simulink model "ltao_e2e"  (R2022b)
settings: Solver=FixedStepDiscrete  StartTime=0.0  StopTime=30  FixedStep=FEM_Ts  MaxStep=FEM_Ts  RelTol=1e-2
InitFcn:
  | %
  | % Initialization callback function
  | %
  | 
  | try
  |    fprintf('\nGMT IMS version (%s)!\n',simulink_fname );
  | 
  |    % Get Simulink model directory
  |    [filepath,name,ext] = fileparts(which(bdroot));
  | 
  |    if ~strcmp(filepath,pwd)
  |       fprintf('\nChanging current directory to \n %s \n',filepath);
  |       cd(filepath);
  |    end
  | 
  |    %
  |  if(osim.bpless_wl)
  |     fprintf('Generating bumpless wind load time series\n');
  |  end
  | catch
  |    warning('Running the InitFcn from puSimulate script');
  | end
values from neighbouring files (symbols this model uses):
  asm_kl_dist = 0*asm_kl_dist    [load_ltao_e2e.m]
  asm_ssG = XiKL' * asm_ssG * XiKL    [load_ltao_e2e.m]
  Cpi_d = eye(n_Zmodes)* c2d(st.asm.fpi, Ts, c2d_opts)    [evalM2asm_modal.m]    (also in load_ltao_e2e.m = c2d(st.asm.fpi, FEM_Ts, c2d_opts))
  fao_d = c2d(st.glao.fao, st.glao.T, c2d_opts)    [evalM2asm_modal.m]    (also in load_ltao_e2e.m = c2d(st.ltao.fao, FEM_Ts, c2d_opts))
  fao_d4k = c2d(st.ltao.fao, 1/4e3, c2d_opts)    [evalM2asm_modal.m]    (also in load_ltao_e2e.m = c2d(st.ltao.fao, FEM_Ts, c2d_opts))
  FEM_Ts = 1/8e3    (= 0.000125)    [load_ltao_e2e.m]
  fes = c2d(tf((fc_es^2)*4*(pi^2),[1, 2*0.8*fc_es*2*pi, (fc_es^2)*4*(pi^2)]),     st.ltao.T,c2d_opts)    [load_ltao_e2e.m]
  flag_1stOdyn_d = tf(c2d(flag(2,1), Ts, c2d_opts))    [evalM2asm_modal.m]    (also in load_ltao_e2e.m = tf(c2d(flag(2,1),FEM_Ts,c2d_opts)))
  flag_2ndOdyn_d = tf(c2d(flag(3,1), Ts, c2d_opts))    [evalM2asm_modal.m]    (also in load_ltao_e2e.m = tf(c2d(flag(3,1),FEM_Ts,c2d_opts)))
  fm2off = c2d(f_ct_m2off, st.ltao.T,c2d_opts)    [load_ltao_e2e.m]
  fpre_d = tf(c2d(st.asm.fpre, Ts, c2d_opts))    [evalM2asm_modal.m]    (also in load_ltao_e2e.m = tf(c2d(fpre,FEM_Ts,c2d_opts)))
  gtt2mnt = eye(2)/(rbm2gtt * Hk_mnt_m1m2)    [load_ltao_e2e.m]
  Hk_mnt_m1m2 = Cm1m2*pinv(Cmnt)    [load_ltao_e2e.m]
  Hpd_d = eye(n_Zmodes)* c2d(st.asm.fpd, Ts, c2d_opts)    [evalM2asm_modal.m]    (also in load_ltao_e2e.m = c2d(st.asm.fpd, FEM_Ts, 'Tustin'))
  K_asm_2_m2p = K_m2p / K_m2p6F_2_asmRB    [load_ltao_e2e.m]
  K_m2p = gainMatrix(out_m2p_mc,in_m2p_mc) -gainMatrix(out_m2p_mc,in_m2p_m2)          - gainMatrix(out_m2p_m2,in_m2p_mc) +gainMatrix(out_m2p_m2,in_m2p_m2)    [load_ltao_e2e.m]
  K_m2p6F_2_asmRB = gainMatrix(out_asm_RB,in_m2p_mc) - gainMatrix(out_asm_RB,in_m2p_m2)    [load_ltao_e2e.m]
  K_m2p_2_asm = K_m2p6F_2_asmRB/ K_m2p    [load_ltao_e2e.m]
  K_m2p_2_es = gainMatrix(out_m2es,in_m2p_mc)-gainMatrix(out_m2es,in_m2p_m2)    [load_ltao_e2e.m]
  Kasmoff = K_asm_2_m2p *         [Kasmoff_{1},Kasmoff_{2},Kasmoff_{3},Kasmoff_{4},         Kasmoff_{5},Kasmoff_{6},Kasmoff_{7}]    [load_ltao_e2e.m]
  Ki_m2off = 1.3    [load_ltao_e2e.m]
  Km1rbm_es = (KhpF2es/KhpF2m1rbm)    [load_ltao_e2e.m]
  Ks = cell(7,1)    [load_ltao_e2e.m]
  m1_rbm_dist = zeros(42,1)    [load_ltao_e2e.m]
  m2_rbm_dist = 0*m2_rbm_dist    [load_ltao_e2e.m]
  m2_rbm_offset = 0*m2_rbm_offset    [load_ltao_e2e.m]
  PG = zeros(length(om2),6)    [evalM2asm_modal.m]    (also in load_ltao_e2e.m)
  phiB = inputs2ModalF(mode_ind_vec,indDesInputs) * KinputT    [load_ltao_e2e.m]
  phiC = KoutputT * modalDisp2Outputs(indDesOutputs,mode_ind_vec)    [load_ltao_e2e.m]
  Psi_ss = KoutputT *gainMatrix(indDesOutputs,indDesInputs)* KinputT - K_ss    [load_ltao_e2e.m]
  Rm2es = pinv(K_asm_2_es, 1e-2)    [load_ltao_e2e.m]
  segPTT2asmCMD = cell(7,1)    [load_ltao_e2e.m]
  st = getcontrol_asm()    [evalM2asm_modal.m]    (also in load_ltao_e2e.m)
  T_pos2e = (K_m2p_2_es / K_m2p)    [load_ltao_e2e.m]
undefined symbols (not defined in the file or in its folder): a, az, az_ff_en, b, c, D_seg_piston, D_seg_tt, DiscIntNeverNeededParam, el, fem, gir, m1sys, m2pos, magnitude, mount, osim, rbm2gtt, Rm1es, sm, VC_modal_stiff
libraries: ims_block_library x7, simulink x2
(part 1 of 3)
settings Model: SimulationMode=accelerator  Creator=RRomano  LastModifiedBy=rromano
settings SolverCC: MaxConsecutiveMinStep=10  ZeroCrossAlgorithm=Adaptive  AlgebraicLoopSolver=TrustRegion
settings DataIOCC: SaveOutput=off  SignalLogging=off  DSMLogging=off  SaveTime=off  ReturnWorkspaceOutputs=off
settings OptimizationCC: DefaultParameterBehavior=Inlined  StrengthReduction=on  PassReuseOutputArgsAs=Individual arguments  EfficientMapNaN2IntZero=off  SimCompilerOptimization=on  AccelVerboseBuild=on  OptimizeBlockOrder=speed  OptimizationPriority=Speed  OptimizationCustomize=off  MultiThreadedLoops=on  EfficientTunableParamExpr=on
settings DebuggingCC: InheritedTsInSrcMsg=none  MultiTaskRateTransMsg=warning  ParameterTunabilityLossMsg=error  UnconnectedInputMsg=warning  UnconnectedOutputMsg=warning  UnconnectedLineMsg=warning  SFUnexpectedBacktrackingDiag=warning  SFNoUnconditionalDefaultTransitionDiag=warning  SFExecutionAtInitializationDiag=none  SFMachineParentedDataDiag=warning  ArithmeticOperatorsInVariantConditions=warning
settings HardwareCC: ProdBitPerLong=64  ProdHWDeviceType=Intel->x86-64 (Linux 64)  TargetBitPerLong=64  TargetBitPerPointer=64  TargetBitPerSizeT=64  TargetBitPerPtrDiffT=64  TargetLongLongMode=on  TargetIntDivRoundTo=Zero  TargetEndianess=LittleEndian  TargetWordSize=64  TargetHWDeviceType=MATLAB Host  ProdEqTarget=off
settings ModelReferenceCC: EnableRefExpFcnMdlSchedulingChecks=on
settings SFSimCC: SimUseLocalCustomCode=off  MATLABDynamicMemAlloc=off  CustomCodeUndefinedFunction=UseInterfaceOnly
settings RTWCC: Description=Embedded Coder  SystemTargetFile=ert.tlc  GenCodeOnly=on  TemplateMakefile=ert_default_tmf  GenerateReport=on  BuildConfiguration=Faster Runs  IncludeHyperlinkInReport=on  GenerateTraceInfo=on  GenerateTraceReport=on  GenerateTraceReportSl=on  GenerateTraceReportSf=on  GenerateTraceReportEml=on  DLArmComputeVersion=19.05
settings CodeAppCC: ForceParamTrailComments=on  IgnoreCustomStorageClasses=off  MaxIdLength=128  OperatorAnnotations=on  SimulinkDataObjDesc=on  SFDataObjDesc=on  InsertBlockDesc=on  MATLABSourceComments=on
settings ERTTargetCC: GenerateSampleERTMain=on  InlinedParameterPlacement=NonHierarchical  ERTCustomFileTemplate=example_file_process.tlc
settings ConfigComp: CovMetricSettings=dw  CovSaveCumulativeToWorkspaceVar=on  CovSaveSingleToWorkspaceVar=on  CovExternalEMLEnable=off

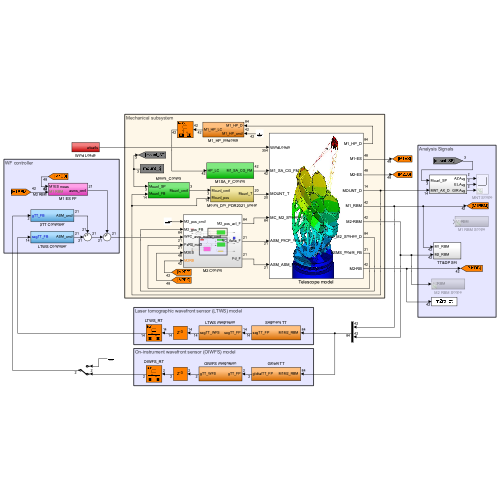
[thumbnail: Simulink's stored preview of the top-level diagram]
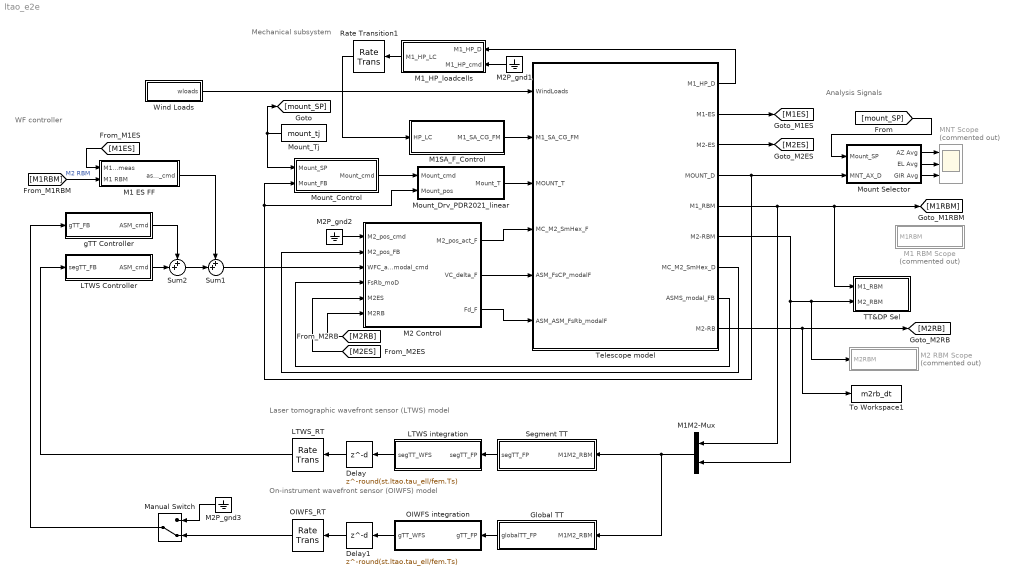
== system ltao_e2e ==
  note: Laser tomographic wavefront sensor (LTWS) model
  note: Analysis Signals
  note: Mechanical subsystem
  note: WF controller
  note: On-instrument wavefront sensor (OIWFS) model
  Delay : Delay  DelayLength=round(st.ltao.tau_ell/fem.Ts)
  Delay1 : Delay  DelayLength=round(st.ltao.tau_ell/fem.Ts)
  Global TT : Subsystem
  LTWS Controller : Subsystem
  LTWS integration : Subsystem
  LTWS_RT : RateTransition  Deterministic=off  OutPortSampleTime=st.ltao.T
  M1 ES FF : Subsystem
  M1 RBM Scope : Subsystem  Commented=on
  M1M2-Mux : Mux  Inputs=[42 42]
  M1SA_F_Control : Subsystem
  M1_HP_loadcells : Subsystem
  M2 Control : Subsystem
  M2 RBM Scope : Subsystem  Commented=on
  M2P_gnd1 : Ground
  M2P_gnd2 : Ground
  M2P_gnd3 : Ground
  MNT Scope : Scope  Commented=on  NumInputPorts=3
  Manual Switch : ManualSwitch  CurrentSetting=0
  Mount Selector : Subsystem
  Mount_Control : Subsystem
  Mount_Drv_PDR2021_linear : Subsystem
  Mount_Tj : FromWorkspace  VariableName=mount_tj  OutputAfterFinalValue=Setting to zero
  OIWFS integration : Subsystem
  OIWFS_RT : RateTransition  Deterministic=off  OutPortSampleTime=st.ltao.T
  Rate Transition1 : RateTransition  Integrity=off  OutPortSampleTime=m1sys{1}.ofl.SSdtC{1}.Ts
  Segment TT : Subsystem
  Sum1 : Sum  Inputs=++|
  Sum2 : Sum  Inputs=++|
  TT&DP Sel : Subsystem
  Telescope model : Subsystem
      mask Display: image('$imagefile'); % Use "Edit Image" on toolstrip to change.
  To Workspace1 : ToWorkspace  VariableName=m2rb_dt  SampleTime=-1
  Wind Loads : Subsystem
  gTT Controller : Subsystem
  wires:
  Mount Selector/1(AZ Avg) -> MNT Scope/1
  Mount Selector/2(EL Avg) -> MNT Scope/2
  Mount Selector/3(GIR Avg) -> MNT Scope/3
  Telescope model/1(M1_HP_D) -> M1_HP_loadcells/1(M1_HP_D)
  M1_HP_loadcells/1(M1_HP_LC) -> Rate Transition1/1
  Mount_Tj/1 -> [mount_SP], Mount_Control/1(Mount_SP)
  [mount_SP] -> Mount Selector/1(Mount_SP)
  M1SA_F_Control/1(M1_SA_CG_FM) -> Telescope model/2(M1_SA_CG_FM)
  Wind Loads/1(wloads) -> Telescope model/1(WindLoads)
  Rate Transition1/1 -> M1SA_F_Control/1(HP_LC)
  Mount_Drv_PDR2021_linear/1(Mount_T) -> Telescope model/3(MOUNT_T)
  Telescope model/4(MOUNT_D) -> Mount Selector/2(MNT_AX_D), Mount_Control/2(Mount_FB), Mount_Drv_PDR2021_linear/2(Mount_pos)
  Mount_Control/1(Mount_cmd) -> Mount_Drv_PDR2021_linear/1(Mount_cmd)
  Telescope model/2(M1-ES) -> [M1ES]
  M2P_gnd1/1 -> M1_HP_loadcells/2(M1_HP_cmd)
  Segment TT/1(segTT_FP) -> LTWS integration/1(segTT_FP)
  LTWS integration/1(segTT_WFS) -> Delay/1
  Telescope model/5(M1_RBM) -> M1M2-Mux/1, TT&DP Sel/1(M1_RBM), [M1RBM]
  LTWS Controller/1(ASM_cmd) -> Sum2/2
  [M1ES] -> M1 ES FF/1(M1ES meas)
  Telescope model/9(M2-RB) -> To Workspace1/1, [M2RB]
  Telescope model/6(M2-RBM) -> M2 RBM Scope/1(M2RBM), TT&DP Sel/2(M2_RBM), M1M2-Mux/2
  OIWFS integration/1(gTT_WFS) -> Delay1/1
  M1M2-Mux/1 -> Segment TT/1("M1M2_RBM "), Global TT/1("M1M2_RBM ")
  Sum2/1 -> Sum1/2
  Global TT/1(globalTT_FP) -> OIWFS integration/1(gTT_FP)
  Delay/1 -> LTWS_RT/1
  gTT Controller/1(ASM_cmd) -> Sum2/1
  Delay1/1 -> OIWFS_RT/1
  LTWS_RT/1 -> LTWS Controller/1(segTT_FB)
  OIWFS_RT/1 -> Manual Switch/2
  Telescope model/3(M2-ES) -> [M2ES]
  M2P_gnd3/1 -> Manual Switch/1
  [M1RBM] -> M1 ES FF/2(M1 RBM)  "M2 RBM"
  Manual Switch/1 -> gTT Controller/1(gTT_FB)
  M2P_gnd2/1 -> M2 Control/1(M2_pos_cmd)
  Telescope model/7(MC_M2_SmHex_D) -> M2 Control/2(M2_pos_FB)
  Telescope model/8(ASMS_modal_FB) -> M2 Control/4(FsRb_moD)
  M2 Control/1(M2_pos_act_F) -> Telescope model/4(MC_M2_SmHex_F)
  M2 Control/2(VC_delta_F) -> Telescope model/5(ASM_FsCP_modalF)
  M2 Control/3(Fd_F) -> Telescope model/6(ASM_ASM_FsRb_modalF)
  [M2ES] -> M2 Control/5(M2ES)
  [M2RB] -> M2 Control/6(M2RB)
  Sum1/1 -> M2 Control/3(WFC_asm_modal_cmd)
  M1 ES FF/1(asms_cmd) -> Sum1/1

== system ltao_e2e/Global TT ==
  "M1M2_RBM " : Inport
  Global TT optical sensitivity matrix : Gain  Gain=rbm2gtt  Multiplication=Matrix(K*u)
  globalTT_FP : Outport  VectorParamsAs1DForOutWhenUnconnected=off
  wires:
  Global TT optical sensitivity matrix/1 -> globalTT_FP/1
  "M1M2_RBM "/1 -> Global TT optical sensitivity matrix/1

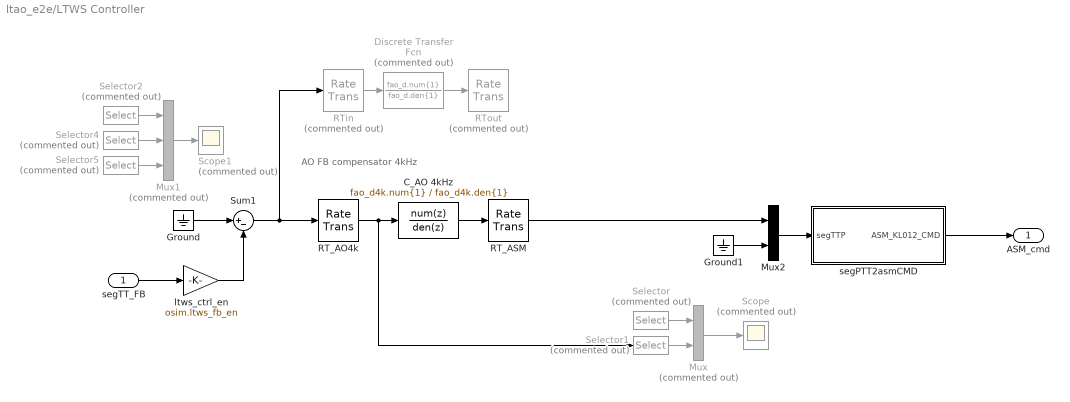
== system ltao_e2e/LTWS Controller ==
  note: AO FB compensator 4kHz
  segTT_FB : Inport  PortDimensions=14
  C_AO 4kHz : DiscreteTransferFcn  Numerator=fao_d4k.num{1}  Denominator=fao_d4k.den{1}  SampleTime=fao_d4k.Ts
  Discrete Transfer Fcn : DiscreteTransferFcn  Commented=on  Numerator=fao_d.num{1}  Denominator=fao_d.den{1}  SampleTime=fao_d.Ts
  Ground : Ground
  Ground1 : Ground
  Mux : Mux  Commented=on  Inputs=2
  Mux1 : Mux  Commented=on  Inputs=3
  Mux2 : Mux  Inputs=[14,7]
  RT_AO4k : RateTransition  Integrity=off  Deterministic=off  OutPortSampleTimeOpt=Inherit
  RT_ASM : RateTransition  Integrity=off  Deterministic=off  OutPortSampleTimeOpt=Inherit
  RTin : RateTransition  Commented=on  Deterministic=off  OutPortSampleTime=fao_d.Ts
  RTout : RateTransition  Commented=on  Integrity=off  Deterministic=off  OutPortSampleTimeOpt=Inherit
  Scope : Scope  Commented=on
  Scope1 : Scope  Commented=on
  Selector{,1..2,4..5} (5 alike) : Selector  Commented=on  InputPortWidth=462  IndexOptions=Index vector (dialog)  Indices=[1 4]  OutputSizes=1
  Sum1 : Sum  Inputs=|+-
  ltws_ctrl_en : Gain  Gain=osim.ltws_fb_en
  segPTT2asmCMD : Subsystem
  ASM_cmd : Outport  VectorParamsAs1DForOutWhenUnconnected=off
  wires:
  Ground/1 -> Sum1/1
  RTin/1 -> Discrete Transfer Fcn/1
  Mux/1 -> Scope/1
  Selector1/1 -> Mux/2
  Selector/1 -> Mux/1
  Discrete Transfer Fcn/1 -> RTout/1
  Sum1/1 -> RTin/1, RT_AO4k/1
  Selector4/1 -> Mux1/2
  Selector2/1 -> Mux1/1
  Selector5/1 -> Mux1/3
  RT_AO4k/1 -> Selector1/1, C_AO 4kHz/1
  C_AO 4kHz/1 -> RT_ASM/1
  Mux1/1 -> Scope1/1
  segTT_FB/1 -> ltws_ctrl_en/1
  RT_ASM/1 -> Mux2/1
  Ground1/1 -> Mux2/2
  Mux2/1 -> segPTT2asmCMD/1(segTTP)
  segPTT2asmCMD/1(ASM_KL012_CMD) -> ASM_cmd/1
  ltws_ctrl_en/1 -> Sum1/2

== system ltao_e2e/LTWS integration ==
  segTT_FP : Inport
  Discrete-Time Integrator : DiscreteIntegrator  gainval=1  ExternalReset=rising  SampleTime=-1  ICPrevOutput=DiscIntNeverNeededParam  ICPrevScaledInput=DiscIntNeverNeededParam
  Mux1 : Mux  Inputs=2
  Pulse Generator : DiscretePulseGenerator  Period=st.ltao.T/fem.Ts  PulseWidth=2  PhaseDelay=1  SampleTime=fem.Ts
  Selector : Selector  InputPortWidth=14  IndexOptions=Index vector (dialog)  Indices=[1:7:14]  OutputSizes=1
  Selector1 : Selector  InputPortWidth=14  IndexOptions=Index vector (dialog)  Indices=[1:7:14]  OutputSizes=1
  TEST Scope : Scope  Commented=on
  wfs_int_gain : Gain  Gain=1/st.ltao.T
  segTT_WFS : Outport
  wires:
  Pulse Generator/1 -> Discrete-Time Integrator/2
  Discrete-Time Integrator/1 -> wfs_int_gain/1
  segTT_FP/1 -> Selector1/1, Discrete-Time Integrator/1
  wfs_int_gain/1 -> segTT_WFS/1, Selector/1
  Mux1/1 -> TEST Scope/1
  Selector/1 -> Mux1/2
  Selector1/1 -> Mux1/1

== system ltao_e2e/M1 ES FF ==
  M1ES meas : Inport
  M1 RBM : Inport  Port=2
  -1 : Gain  Gain=-1
  ES FF filter : DiscreteFilter  Numerator=fes.num{1}  Denominator=fes.den{1}  SampleTime=fes.Ts  a0EqualsOne=on
  M1ES Reconstructor : Gain  Gain=-Rm1es  Multiplication=Matrix(K*u)
  M1RBM to segPiston : Gain  Gain=D_seg_piston(:,1:42)  Multiplication=Matrix(K*u)
  M1RBM to segTT : Gain  Gain=D_seg_tt(:,1:42)  Multiplication=Matrix(K*u)
  M2P_gnd : Ground
  Manual Switch : ManualSwitch  CurrentSetting=0
  Manual Switch1 : ManualSwitch  CurrentSetting=0
  Mux2 : Mux  Inputs=[14,7]
  RT_M1ES : RateTransition  Deterministic=off
  Rate Transition : RateTransition  Commented=through  Deterministic=off  OutPortSampleTime=st.ltao.T
  Selector : Selector  Commented=through  InputPortWidth=21  IndexOptions=Index vector (dialog)  Indices=15:21  OutputSizes=1
  Selector1 : Selector  Commented=on  InputPortWidth=21  IndexOptions=Index vector (dialog)  Indices=1:3:21  OutputSizes=1
  asmKL0_cmd : Scope  Commented=on
  gPfilter : Gain  Commented=through  Gain=(eye(7) - kron(ones(7),1/7))  Multiplication=Matrix(K*u)
  gTTfilter : Gain  Commented=through  Gain=(eye(14) - kron(eye(2),kron(ones(7),1/7)))  Multiplication=Matrix(K*u)
  segP-M1 Scope : Scope  Commented=on
  segPTT2asmCMD : Subsystem
  asms_cmd : Outport
  wires:
  M1ES meas/1 -> M1ES Reconstructor/1  "M1ES measurements"
  Mux2/1 -> Selector/1, segPTT2asmCMD/1(segTTP)
  M1 RBM/1 -> -1/1  "M1 RBM"
  Manual Switch/1 -> Rate Transition/1
  segPTT2asmCMD/1(ASM_KL012_CMD) -> Manual Switch1/2, Selector1/1
  Selector/1 -> segP-M1 Scope/1
  Selector1/1 -> asmKL0_cmd/1
  M1ES Reconstructor/1 -> Manual Switch/2
  -1/1 -> Manual Switch/1
  Manual Switch1/1 -> RT_M1ES/1
  M2P_gnd/1 -> Manual Switch1/1
  RT_M1ES/1 -> asms_cmd/1
  Rate Transition/1 -> ES FF filter/1
  M1RBM to segTT/1 -> gTTfilter/1
  M1RBM to segPiston/1 -> gPfilter/1
  gTTfilter/1 -> Mux2/1
  gPfilter/1 -> Mux2/2
  ES FF filter/1 -> M1RBM to segPiston/1, M1RBM to segTT/1

== system ltao_e2e/M1 RBM Scope ==
  note: Local motion of M1 segments (in m and rad)
  M1RBM : Inport
  M1 RBM scope : Scope  Commented=on  NumInputPorts=6
  Selector : Selector  InputPortWidth=42  IndexOptions=Index vector (dialog)  Indices=[1:6:42]  OutputSizes=1
  Selector1 : Selector  InputPortWidth=42  IndexOptions=Index vector (dialog)  Indices=[2:6:42]  OutputSizes=1
  Selector2 : Selector  InputPortWidth=42  IndexOptions=Index vector (dialog)  Indices=[3:6:42]  OutputSizes=1
  Selector3 : Selector  InputPortWidth=42  IndexOptions=Index vector (dialog)  Indices=[4:6:42]  OutputSizes=1
  Selector4 : Selector  InputPortWidth=42  IndexOptions=Index vector (dialog)  Indices=[5:6:42]  OutputSizes=1
  Selector5 : Selector  InputPortWidth=42  IndexOptions=Index vector (dialog)  Indices=[6:6:42]  OutputSizes=1
  wires:
  M1RBM/1 -> Selector3/1, Selector4/1, Selector5/1, Selector/1, Selector1/1, Selector2/1
  Selector/1 -> M1 RBM scope/1
  Selector1/1 -> M1 RBM scope/2
  Selector2/1 -> M1 RBM scope/3
  Selector3/1 -> M1 RBM scope/4
  Selector4/1 -> M1 RBM scope/5
  Selector5/1 -> M1 RBM scope/6

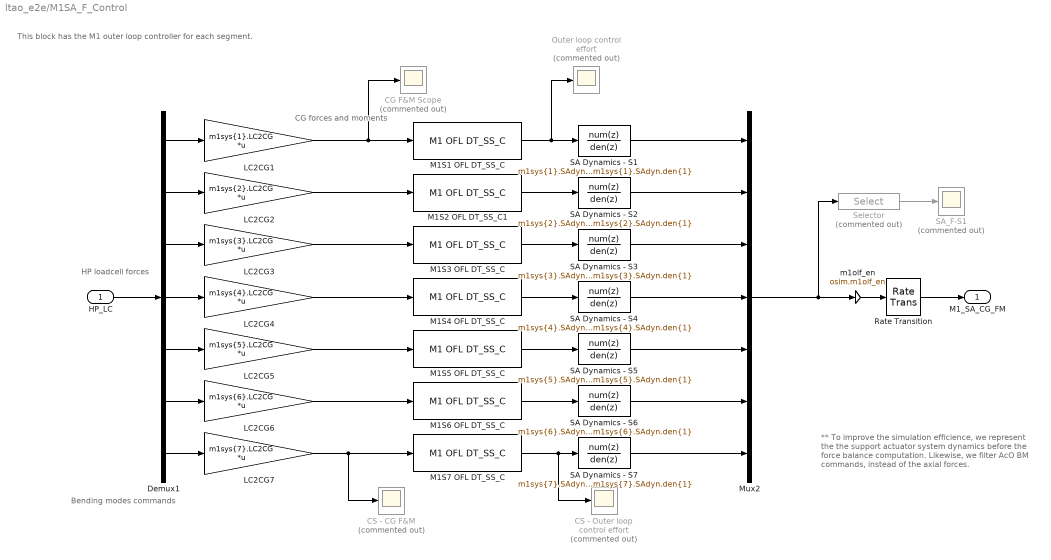
== system ltao_e2e/M1SA_F_Control ==
  note: HP loadcell forces
  note: This block has the M1 outer loop controller for each segment.
  note: CG forces
      | and moments
  note: Bending modes
      | commands
  note: ** To improve the simulation efficience, we represent the the support actuator system dynamics before the force balance computation. Likewise, we filter AcO BM commands, instead of the axial forces.
  HP_LC : Inport
  CG F&M Scope : Scope  Commented=on
  CS - CG F&M : Scope  Commented=on
  CS - Outer loop control effort : Scope  Commented=on
  Demux1 : Demux  Outputs=6*ones(7,1)
  LC2CG1 : Gain  Gain=m1sys{1}.LC2CG  Multiplication=Matrix(K*u)
  LC2CG2 : Gain  Gain=m1sys{2}.LC2CG  Multiplication=Matrix(K*u)
  LC2CG3 : Gain  Gain=m1sys{3}.LC2CG  Multiplication=Matrix(K*u)
  LC2CG4 : Gain  Gain=m1sys{4}.LC2CG  Multiplication=Matrix(K*u)
  LC2CG5 : Gain  Gain=m1sys{5}.LC2CG  Multiplication=Matrix(K*u)
  LC2CG6 : Gain  Gain=m1sys{6}.LC2CG  Multiplication=Matrix(K*u)
  LC2CG7 : Gain  Gain=m1sys{7}.LC2CG  Multiplication=Matrix(K*u)
  M1S1 OFL DT_SS_C : ims_block_library/M1 OFL DT_SS_C  dt_SS_struct=m1sys{1}.ofl.SSdtC
  M1S2 OFL DT_SS_C1 : ims_block_library/M1 OFL DT_SS_C  dt_SS_struct=m1sys{2}.ofl.SSdtC
  M1S3 OFL DT_SS_C : ims_block_library/M1 OFL DT_SS_C  dt_SS_struct=m1sys{3}.ofl.SSdtC
  M1S4 OFL DT_SS_C : ims_block_library/M1 OFL DT_SS_C  dt_SS_struct=m1sys{4}.ofl.SSdtC
  M1S5 OFL DT_SS_C : ims_block_library/M1 OFL DT_SS_C  dt_SS_struct=m1sys{5}.ofl.SSdtC
  M1S6 OFL DT_SS_C : ims_block_library/M1 OFL DT_SS_C  dt_SS_struct=m1sys{6}.ofl.SSdtC
  M1S7 OFL DT_SS_C : ims_block_library/M1 OFL DT_SS_C  dt_SS_struct=m1sys{7}.ofl.SSdtC
  Mux2 : Mux  Inputs=7
  Outer loop control effort : Scope  Commented=on
  Rate Transition : RateTransition  Integrity=off  OutPortSampleTime=FEM_Ts
  SA Dynamics - S1 : DiscreteTransferFcn  Numerator=m1sys{1}.SAdyn.num{1}  Denominator=m1sys{1}.SAdyn.den{1}  SampleTime=m1sys{1}.ofl.Ts  a0EqualsOne=on
  SA Dynamics - S2 : DiscreteTransferFcn  Numerator=m1sys{2}.SAdyn.num{1}  Denominator=m1sys{2}.SAdyn.den{1}  SampleTime=m1sys{1}.ofl.SSdtC{1}.Ts  a0EqualsOne=on
  SA Dynamics - S3 : DiscreteTransferFcn  Numerator=m1sys{3}.SAdyn.num{1}  Denominator=m1sys{3}.SAdyn.den{1}  SampleTime=m1sys{1}.ofl.SSdtC{1}.Ts  a0EqualsOne=on
  SA Dynamics - S4 : DiscreteTransferFcn  Numerator=m1sys{4}.SAdyn.num{1}  Denominator=m1sys{4}.SAdyn.den{1}  SampleTime=m1sys{1}.ofl.SSdtC{1}.Ts  a0EqualsOne=on
  SA Dynamics - S5 : DiscreteTransferFcn  Numerator=m1sys{5}.SAdyn.num{1}  Denominator=m1sys{5}.SAdyn.den{1}  SampleTime=m1sys{1}.ofl.SSdtC{1}.Ts  a0EqualsOne=on
  SA Dynamics - S6 : DiscreteTransferFcn  Numerator=m1sys{6}.SAdyn.num{1}  Denominator=m1sys{6}.SAdyn.den{1}  SampleTime=m1sys{1}.ofl.SSdtC{1}.Ts  a0EqualsOne=on
  SA Dynamics - S7 : DiscreteTransferFcn  Numerator=m1sys{7}.SAdyn.num{1}  Denominator=m1sys{7}.SAdyn.den{1}  SampleTime=m1sys{1}.ofl.SSdtC{1}.Ts  a0EqualsOne=on
  SA_F-S1 : Scope  Commented=on
  Selector : Selector  Commented=on  InputPortWidth=2316  IndexOptions=Index vector (dialog)  Indices=[1:335]  OutputSizes=1
  m1olf_en : Gain  Gain=osim.m1olf_en
  M1_SA_CG_FM : Outport  VectorParamsAs1DForOutWhenUnconnected=off
  wires:
  HP_LC/1 -> Demux1/1
  M1S1 OFL DT_SS_C/1 -> Outer loop control effort/1, SA Dynamics - S1/1
  M1S2 OFL DT_SS_C1/1 -> SA Dynamics - S2/1
  M1S3 OFL DT_SS_C/1 -> SA Dynamics - S3/1
  M1S4 OFL DT_SS_C/1 -> SA Dynamics - S4/1
  M1S5 OFL DT_SS_C/1 -> SA Dynamics - S5/1
  M1S6 OFL DT_SS_C/1 -> SA Dynamics - S6/1
  M1S7 OFL DT_SS_C/1 -> CS - Outer loop control effort/1, SA Dynamics - S7/1
  LC2CG7/1 -> M1S7 OFL DT_SS_C/1, CS - CG F&M/1
  LC2CG6/1 -> M1S6 OFL DT_SS_C/1
  LC2CG5/1 -> M1S5 OFL DT_SS_C/1
  LC2CG4/1 -> M1S4 OFL DT_SS_C/1
  LC2CG3/1 -> M1S3 OFL DT_SS_C/1
  LC2CG2/1 -> M1S2 OFL DT_SS_C1/1
  LC2CG1/1 -> M1S1 OFL DT_SS_C/1, CG F&M Scope/1
  Demux1/1 -> LC2CG1/1
  Demux1/2 -> LC2CG2/1
  Demux1/3 -> LC2CG3/1
  Demux1/4 -> LC2CG4/1
  Demux1/5 -> LC2CG5/1
  Demux1/6 -> LC2CG6/1
  Demux1/7 -> LC2CG7/1
  Mux2/1 -> m1olf_en/1, Selector/1
  Selector/1 -> SA_F-S1/1
  SA Dynamics - S1/1 -> Mux2/1
  SA Dynamics - S2/1 -> Mux2/2
  SA Dynamics - S3/1 -> Mux2/3
  SA Dynamics - S4/1 -> Mux2/4
  SA Dynamics - S5/1 -> Mux2/5
  SA Dynamics - S6/1 -> Mux2/6
  SA Dynamics - S7/1 -> Mux2/7
  m1olf_en/1 -> Rate Transition/1
  Rate Transition/1 -> M1_SA_CG_FM/1

== system ltao_e2e/M1_HP_loadcells ==
  note: This block converts from CG displacements and rotations,
      | and converts to Hard Point lengths.  Hard point lengths are
      | changed by applying an equal and opposite force to the hard
      | point, and then offseting output by the commanded change
      | in position.
  note: Hexapod Offset Forces
  note: LC Forces (N)
  M1_HP_D : Inport
  M1_HP_cmd : Inport  Port=2
  Demux1 : Demux  Outputs=6*ones(7,1)
  Demux2 : Demux  Outputs=6*ones(14,1);%6*ones(7,1)
  M1S1 Loadcell : Subsystem
  M1S2 Loadcell : Subsystem
  M1S3 Loadcell : Subsystem
  M1S4 Loadcell : Subsystem
  M1S5 Loadcell : Subsystem
  M1S6 Loadcell : Subsystem
  M1S7 Control : Subsystem
  Mux2 : Mux  Inputs=7
  Scope : Scope  NumInputPorts=2
  M1_HP_LC : Outport  VectorParamsAs1DForOutWhenUnconnected=off
  wires:
  Demux2/9 -> M1S5 Loadcell/2(HP_D_cell)
  Demux2/3 -> M1S2 Loadcell/2(HP_D_cell)
  Demux2/5 -> M1S3 Loadcell/2(HP_D_cell)
  Demux2/13 -> M1S7 Control/2(HP_D_cell)
  Demux2/11 -> M1S6 Loadcell/2(HP_D_cell)
  Demux2/4 -> M1S2 Loadcell/3(HP_D_face)
  Demux2/6 -> M1S3 Loadcell/3(HP_D_face)
  Demux2/10 -> M1S5 Loadcell/3(HP_D_face)
  Demux2/12 -> M1S6 Loadcell/3(HP_D_face)
  Demux2/14 -> M1S7 Control/3(HP_D_face)
  M1_HP_D/1 -> Demux2/1
  M1S1 Loadcell/1(HP_F_meas) -> Mux2/1
  M1S2 Loadcell/1(HP_F_meas) -> Mux2/2
  M1S3 Loadcell/1(HP_F_meas) -> Mux2/3
  M1S5 Loadcell/1(HP_F_meas) -> Mux2/5
  M1S6 Loadcell/1(HP_F_meas) -> Mux2/6
  M1S7 Control/1(HP_F_meas) -> Mux2/7
  Demux2/2 -> M1S1 Loadcell/3(HP_D_face)
  Demux2/1 -> M1S1 Loadcell/2(HP_D_cell)
  M1S4 Loadcell/1(HP_F_meas) -> Mux2/4
  Demux2/7 -> M1S4 Loadcell/2(HP_D_cell)
  Demux2/8 -> M1S4 Loadcell/3(HP_D_face)
  M1_HP_cmd/1 -> Demux1/1
  Demux1/1 -> Scope/1, M1S1 Loadcell/1(HP_F_cmd)
  Demux1/2 -> Scope/2, M1S2 Loadcell/1(HP_F_cmd)
  Demux1/3 -> M1S3 Loadcell/1(HP_F_cmd)
  Demux1/4 -> M1S4 Loadcell/1(HP_F_cmd)
  Demux1/5 -> M1S5 Loadcell/1(HP_F_cmd)
  Demux1/6 -> M1S6 Loadcell/1(HP_F_cmd)
  Demux1/7 -> M1S7 Control/1(HP_F_cmd)
  Mux2/1 -> M1_HP_LC/1

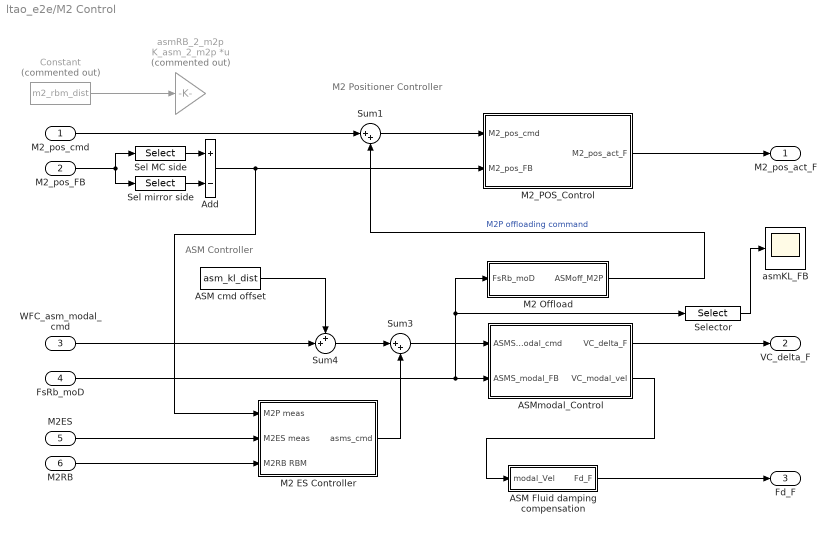
== system ltao_e2e/M2 Control ==
  note: ASM Controller
  note: M2 Positioner Controller
  M2_pos_cmd : Inport
  M2_pos_FB : Inport  Port=2
  WFC_asm_modal_cmd : Inport  Port=3
  FsRb_moD : Inport  Port=4
  M2ES : Inport  Port=5
  M2RB : Inport  Port=6
  ASM Fluid damping compensation : Subsystem
  ASM cmd offset : Constant  Value=asm_kl_dist
  ASMmodal_Control : Subsystem
  Add : Sum  Inputs=+-
  Constant : Constant  Commented=on  Value=m2_rbm_dist
  M2 ES Controller : Subsystem
  M2 Offload : Subsystem
      settings: PortSchema="{\"entries\":[{\"content\":{\"sides\":[{\"content\":{\"connectorIds\":[]},\"type\":\"ConnectorPlacement.EquallySpacedRectSide\",\"uuid\":\"80c6d432-68b0-4374-a7c7-9aefa5201820\"},{\"content\":{\"connectorIds\":[],\"side\":\"RIGHT\"},\"type\":\"ConnectorPlacement.EquallySpacedRectSide\",\"uuid\":\"9786590d-3c3b-41fe-8a5d-655d749c782c\"},{\"content\":{\"connectorIds\":[\"Out1\"],\"side\":\"TOP\"},\"type\":\"ConnectorPlacement.EquallySpacedRectSide\",\"uuid\":\"175f9168-078a-41fa-a182-5172074c41bc\"},{\"content\":{\"connectorIds\":[\"In1\"],\"side\":\"BOTTOM\"},\"type\":\"ConnectorPlacement.EquallySpacedRectSide\",\"uuid\":\"067ec6fa-f778-428a-bcb3-24cbcc4d1ba2\"}]},\"type\":\"ConnectorPlacement.EquallySpacedConnector\",\"uuid\":\"b29ad644-530a-4261-9691-cce7a2457dbe\"}],\"packageUris\":[\"http://schema.mathworks.com/mf0/Connector/R2020b\"],\"version\":\"1.0\"}"
  M2_POS_Control : Subsystem
  Sel MC side : Selector  InputPortWidth=84  IndexOptions=Index vector (dialog)  Indices=[1:2:84]  OutputSizes=1
  Sel mirror side : Selector  InputPortWidth=84  IndexOptions=Index vector (dialog)  Indices=[2:2:84]  OutputSizes=1
  Selector : Selector  InputPortWidth=21  IndexOptions=Index vector (dialog)  Indices=[1:3,19:21]  OutputSizes=1
  Sum1 : Sum  Inputs=|++
  Sum3 : Sum  Inputs=|++
  Sum4 : Sum  Inputs=++|
  asmKL_FB : Scope
  asmRB_2_m2p : Gain  Commented=on  Gain=K_asm_2_m2p  Multiplication=Matrix(K*u)
  M2_pos_act_F : Outport
  VC_delta_F : Outport  Port=2
  Fd_F : Outport  Port=3
  wires:
  M2_POS_Control/1(M2_pos_act_F) -> M2_pos_act_F/1
  FsRb_moD/1 -> Selector/1, M2 Offload/1(FsRb_moD), ASMmodal_Control/2(ASMS_modal_FB)
  ASM Fluid damping compensation/1(Fd_F) -> Fd_F/1
  ASMmodal_Control/2(VC_modal_vel) -> ASM Fluid damping compensation/1(modal_Vel)
  ASMmodal_Control/1(VC_delta_F) -> VC_delta_F/1
  M2 Offload/1(ASMoff_M2P) -> Sum1/2  "M2P offloading command"
  M2ES/1 -> M2 ES Controller/2(M2ES meas)
  M2RB/1 -> M2 ES Controller/3(M2RB RBM)
  Sum1/1 -> M2_POS_Control/1(M2_pos_cmd)
  Sum4/1 -> Sum3/1
  M2 ES Controller/1(asms_cmd) -> Sum3/2
  ASM cmd offset/1 -> Sum4/1
  WFC_asm_modal_cmd/1 -> Sum4/2
  M2_pos_cmd/1 -> Sum1/1
  Sum3/1 -> ASMmodal_Control/1(ASMS_modal_cmd)
  Selector/1 -> asmKL_FB/1
  Constant/1 -> asmRB_2_m2p/1
  Add/1 -> M2 ES Controller/1(M2P meas), M2_POS_Control/2(M2_pos_FB)
  Sel mirror side/1 -> Add/2
  Sel MC side/1 -> Add/1
  M2_pos_FB/1 -> Sel mirror side/1, Sel MC side/1

== system ltao_e2e/M2 RBM Scope ==
  note: Local motion of M2 segments (in m and rad)
  M2RBM : Inport
  M2 RBM scope : Scope  NumInputPorts=6
  Selector : Selector  InputPortWidth=42  IndexOptions=Index vector (dialog)  Indices=[1:6:42]  OutputSizes=1
  Selector1 : Selector  InputPortWidth=42  IndexOptions=Index vector (dialog)  Indices=[2:6:42]  OutputSizes=1
  Selector2 : Selector  InputPortWidth=42  IndexOptions=Index vector (dialog)  Indices=[3:6:42]  OutputSizes=1
  Selector3 : Selector  InputPortWidth=42  IndexOptions=Index vector (dialog)  Indices=[4:6:42]  OutputSizes=1
  Selector4 : Selector  InputPortWidth=42  IndexOptions=Index vector (dialog)  Indices=[5:6:42]  OutputSizes=1
  Selector5 : Selector  InputPortWidth=42  IndexOptions=Index vector (dialog)  Indices=[6:6:42]  OutputSizes=1
  wires:
  M2RBM/1 -> Selector3/1, Selector4/1, Selector5/1, Selector/1, Selector1/1, Selector2/1
  Selector/1 -> M2 RBM scope/1
  Selector1/1 -> M2 RBM scope/2
  Selector2/1 -> M2 RBM scope/3
  Selector3/1 -> M2 RBM scope/4
  Selector4/1 -> M2 RBM scope/5
  Selector5/1 -> M2 RBM scope/6

== system ltao_e2e/Mount Selector ==
  note: Motion in rad
  Mount_SP : Inport
  MNT_AX_D : Inport  Port=2
  Demux1 : Demux  Outputs=[1,1,1]
  Demux3 : Demux  Outputs=3
  Drv_Pos_avg : Gain  Gain=blkdiag(1/4*ones(1,4),1/6*ones(1,6),1/4*ones(1,4))  Multiplication=Matrix(K*u) (u vector)
  Mux : Mux  Inputs=2
  Mux1 : Mux  Inputs=2
  Mux2 : Mux  Inputs=2
  To Workspace2 : ToWorkspace  VariableName=mnt_dt  SampleTime=-1
  AZ Avg : Outport  VectorParamsAs1DForOutWhenUnconnected=off
  EL Avg : Outport  Port=2  VectorParamsAs1DForOutWhenUnconnected=off
  GIR Avg : Outport  Port=3  VectorParamsAs1DForOutWhenUnconnected=off
  wires:
  MNT_AX_D/1 -> Drv_Pos_avg/1
  Mux/1 -> AZ Avg/1
  Demux3/1 -> Mux/2
  Mux1/1 -> EL Avg/1
  Demux3/2 -> Mux1/2
  Demux3/3 -> Mux2/2
  Mux2/1 -> GIR Avg/1
  Mount_SP/1 -> Demux1/1
  Demux1/3 -> Mux2/1
  Demux1/1 -> Mux/1
  Demux1/2 -> Mux1/1
  Drv_Pos_avg/1 -> To Workspace2/1, Demux3/1

== system ltao_e2e/Mount_Control ==
  note: Feedback controller
  note: Feedforward controller
  note: Notes :
      | 1) These loops consider the average of the mount encoders as feedback signals.
      | 2) The controller outputs are in torque units (Nm).
  Mount_SP : Inport
  Mount_FB : Inport  Port=2
  AZ FB controller : DiscreteStateSpace  A=mount.az.SSdtHfb.A  B=mount.az.SSdtHfb.B  C=mount.az.SSdtHfb.C  D=mount.az.SSdtHfb.D  SampleTime=mount.az.SSdtHfb.Ts
  AZ FF controller : DiscreteStateSpace  A=mount.az.SSdtHff.A  B=mount.az.SSdtHff.B  C=mount.az.SSdtHff.C  D=mount.az.SSdtHff.D  SampleTime=mount.az.SSdtHff.Ts
  DT_siso_SS : Subsystem  Commented=on
  Demux1 : Demux  Outputs=[1,1,1]
  Demux5 : Demux  Outputs=3
  Drv_Pos_avg : Gain  Gain=blkdiag(1/4*ones(1,4),1/6*ones(1,6),1/4*ones(1,4))  Multiplication=Matrix(K*u) (u vector)
  EL FB controller : DiscreteStateSpace  A=mount.el.SSdtHfb.A  B=mount.el.SSdtHfb.B  C=mount.el.SSdtHfb.C  D=mount.el.SSdtHfb.D  SampleTime=mount.el.SSdtHfb.Ts
  EL FF controller : DiscreteStateSpace  A=mount.el.SSdtHff.A  B=mount.el.SSdtHff.B  C=mount.el.SSdtHff.C  D=mount.el.SSdtHff.D  SampleTime=mount.el.SSdtHff.Ts
  GIR FB controller : DiscreteStateSpace  A=mount.gir.SSdtHfb.A  B=mount.gir.SSdtHfb.B  C=mount.gir.SSdtHfb.C  D=mount.gir.SSdtHfb.D  SampleTime=mount.gir.SSdtHfb.Ts
  GIR FF controller : DiscreteStateSpace  A=mount.gir.SSdtHff.A  B=mount.gir.SSdtHff.B  C=mount.gir.SSdtHff.C  D=mount.gir.SSdtHff.D  SampleTime=mount.gir.SSdtHff.Ts
  GIR_adj : Gain  Commented=through  Gain=1.4791
  Mount cmds (Nm) : Scope  Commented=on  NumInputPorts=3
  Mux1 : Mux  Inputs=[1,1,1]
  Mux3 : Mux  Inputs=[1,1,1]
  Sum : Sum  Inputs=|+-
  Sum1 : Sum  Inputs=|+-
  Sum2 : Sum  Inputs=++|
  Sum4 : Sum  Inputs=|+-
  az_ff_en : Gain  Commented=through  Gain=az_ff_en
  Mount_cmd : Outport  VectorParamsAs1DForOutWhenUnconnected=off
  wires:
  Mount_FB/1 -> Drv_Pos_avg/1
  Sum1/1 -> AZ FB controller/1
  Demux1/3 -> Sum4/1, GIR FF controller/1
  Mount_SP/1 -> Demux1/1
  Demux1/2 -> Sum/1, EL FF controller/1
  Sum/1 -> EL FB controller/1
  AZ FF controller/1 -> Mux1/1
  EL FF controller/1 -> Mux1/2
  Mux3/1 -> Sum2/2
  Sum2/1 -> Mount_cmd/1
  GIR FF controller/1 -> Mux1/3
  AZ FB controller/1 -> Mux3/1
  EL FB controller/1 -> Mux3/2
  Mux1/1 -> az_ff_en/1
  Sum4/1 -> GIR_adj/1
  GIR FB controller/1 -> Mux3/3
  Demux5/3 -> Sum4/2
  az_ff_en/1 -> Sum2/1
  Demux1/1 -> Sum1/1, AZ FF controller/1
  Drv_Pos_avg/1 -> Demux5/1
  Demux5/2 -> Sum/2
  Demux5/1 -> Sum1/2
  GIR_adj/1 -> GIR FB controller/1

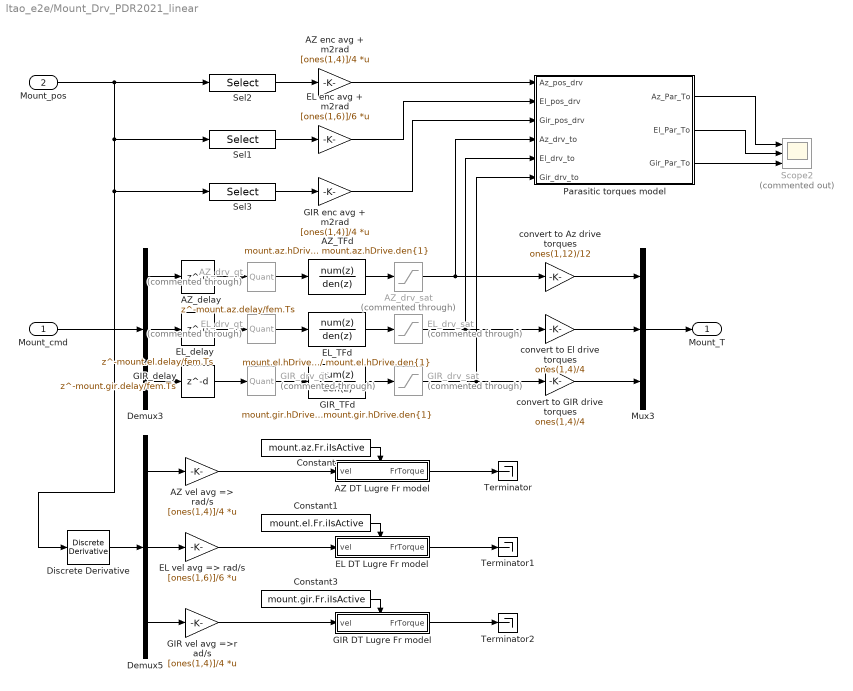
== system ltao_e2e/Mount_Drv_PDR2021_linear ==
  Mount_cmd : Inport
  Mount_pos : Inport  Port=2
  AZ DT Lugre Fr model : Subsystem  TreatAsAtomicUnit=on  mask{frParStruct=mount.az.Fr}
      mask prompts: frParStruct "Structure with the Friction model parameters"
  AZ enc avg + m2rad : Gain  Gain=[ones(1,4)]/4  Multiplication=Matrix(K*u)
  AZ vel avg => rad/s : Gain  Gain=[ones(1,4)]/4  Multiplication=Matrix(K*u)
  AZ_TFd : DiscreteTransferFcn  Numerator=mount.az.hDrive.num{1}  Denominator=mount.az.hDrive.den{1}  SampleTime=mount.el.hDrive.Ts  a0EqualsOne=on
  AZ_delay : Delay  DelayLength=mount.az.delay/fem.Ts  UseCircularBuffer=on  SampleTime=mount.az.hDrive.Ts
  AZ_drv_qt : Quantizer  Commented=through  QuantizationInterval=mount.az.driveQuant
  AZ_drv_sat : Saturate  Commented=through  UpperLimit=mount.az.Tmax  LowerLimit=-mount.az.Tmax
  Constant : Constant  Value=mount.az.Fr.iIsActive
  Constant1 : Constant  Value=mount.el.Fr.iIsActive
  Constant3 : Constant  Value=mount.gir.Fr.iIsActive
  Demux3 : Demux  Outputs=3
  Demux5 : Demux  Outputs=[4,6,4]
  Discrete Derivative : simulink/Discrete/Discrete Derivative  gainval=1  ICPrevScaledInput=0.0  OutMin=[]  OutMax=[]  OutDataType=fixdt(1, 16)  OutScaling=2^-10  DoSatur=off
  EL DT Lugre Fr model : Subsystem  TreatAsAtomicUnit=on  mask{frParStruct=mount.el.Fr}
      mask prompts: frParStruct "Structure with the Friction model parameters"
  EL enc avg + m2rad : Gain  Gain=[ones(1,6)]/6  Multiplication=Matrix(K*u)
  EL vel avg => rad/s : Gain  Gain=[ones(1,6)]/6  Multiplication=Matrix(K*u)
  EL_TFd : DiscreteTransferFcn  Numerator=mount.el.hDrive.num{1}  Denominator=mount.el.hDrive.den{1}  SampleTime=mount.el.hDrive.Ts  a0EqualsOne=on
  EL_delay : Delay  DelayLength=mount.el.delay/fem.Ts  UseCircularBuffer=on  SampleTime=mount.el.hDrive.Ts
  EL_drv_qt : Quantizer  Commented=through  QuantizationInterval=mount.el.driveQuant
  EL_drv_sat : Saturate  Commented=through  UpperLimit=mount.el.Tmax  LowerLimit=-mount.el.Tmax
  GIR DT Lugre Fr model : Subsystem  TreatAsAtomicUnit=on  mask{frParStruct=mount.gir.Fr}
      mask prompts: frParStruct "Structure with the Friction model parameters"
  GIR enc avg + m2rad : Gain  Gain=[ones(1,4)]/4  Multiplication=Matrix(K*u)
  GIR vel avg =>r ad/s : Gain  Gain=[ones(1,4)]/4  Multiplication=Matrix(K*u)
  GIR_TFd : DiscreteTransferFcn  Numerator=mount.gir.hDrive.num{1}  Denominator=mount.gir.hDrive.den{1}  SampleTime=mount.gir.hDrive.Ts  a0EqualsOne=on
  GIR_delay : Delay  DelayLength=mount.gir.delay/fem.Ts  UseCircularBuffer=on  SampleTime=mount.gir.hDrive.Ts
  GIR_drv_qt : Quantizer  Commented=through  QuantizationInterval=mount.gir.driveQuant
  GIR_drv_sat : Saturate  Commented=through  UpperLimit=mount.gir.Tmax  LowerLimit=-mount.gir.Tmax
  Mux3 : Mux  Inputs=[12,4,4]
  "Parasitic torques model " : Subsystem
  Scope2 : Scope  Commented=on  NumInputPorts=3
  Sel1 : Selector  InputPortWidth=14  IndexOptions=Index vector (dialog)  Indices=[5:10]  OutputSizes=1
  Sel2 : Selector  InputPortWidth=14  IndexOptions=Index vector (dialog)  Indices=[1:4]  OutputSizes=1
  Sel3 : Selector  InputPortWidth=14  IndexOptions=Index vector (dialog)  Indices=[11:14]  OutputSizes=1
  Terminator : Terminator
  Terminator1 : Terminator
  Terminator2 : Terminator
  convert to Az drive torques : Gain  Gain=ones(1,12)/12
  convert to El drive torques : Gain  Gain=ones(1,4)/4
  convert to GIR drive torques : Gain  Gain=ones(1,4)/4
  Mount_T : Outport  VectorParamsAs1DForOutWhenUnconnected=off
  wires:
  EL_TFd/1 -> EL_drv_sat/1
  AZ_TFd/1 -> AZ_drv_sat/1
  Mux3/1 -> Mount_T/1
  convert to Az drive torques/1 -> Mux3/1
  convert to El drive torques/1 -> Mux3/2
  convert to GIR drive torques/1 -> Mux3/3
  Demux3/2 -> EL_delay/1
  Demux3/1 -> AZ_delay/1
  AZ_delay/1 -> AZ_drv_qt/1
  EL_delay/1 -> EL_drv_qt/1
  AZ_drv_qt/1 -> AZ_TFd/1
  EL_drv_qt/1 -> EL_TFd/1
  Demux5/1 -> AZ vel avg => rad/s/1
  Demux5/2 -> EL vel avg => rad/s/1
  Demux5/3 -> GIR vel avg =>r ad/s/1
  Discrete Derivative/1 -> Demux5/1
  AZ vel avg => rad/s/1 -> AZ DT Lugre Fr model/1(vel)
  Constant/1 -> AZ DT Lugre Fr model/Enable
  Sel2/1 -> AZ enc avg + m2rad/1
  Sel1/1 -> EL enc avg + m2rad/1
  Mount_pos/1 -> Sel2/1, Discrete Derivative/1, Sel3/1, Sel1/1
  Demux3/3 -> GIR_delay/1
  GIR_TFd/1 -> GIR_drv_sat/1
  GIR_delay/1 -> GIR_drv_qt/1
  GIR_drv_qt/1 -> GIR_TFd/1
  Constant3/1 -> GIR DT Lugre Fr model/Enable
  Sel3/1 -> GIR enc avg + m2rad/1
  AZ enc avg + m2rad/1 -> "Parasitic torques model "/1(Az_pos_drv)
  EL enc avg + m2rad/1 -> "Parasitic torques model "/2(El_pos_drv)
  GIR enc avg + m2rad/1 -> "Parasitic torques model "/3(Gir_pos_drv)
  AZ_drv_sat/1 -> convert to Az drive torques/1, "Parasitic torques model "/4(Az_drv_to)
  EL_drv_sat/1 -> convert to El drive torques/1, "Parasitic torques model "/5(El_drv_to)
  GIR_drv_sat/1 -> convert to GIR drive torques/1, "Parasitic torques model "/6(Gir_drv_to)
  Constant1/1 -> EL DT Lugre Fr model/Enable
  GIR vel avg =>r ad/s/1 -> GIR DT Lugre Fr model/1(vel)
  "Parasitic torques model "/1(Az_Par_To) -> Scope2/1
  "Parasitic torques model "/2(El_Par_To) -> Scope2/2
  "Parasitic torques model "/3(Gir_Par_To) -> Scope2/3
  EL vel avg => rad/s/1 -> EL DT Lugre Fr model/1(vel)
  Mount_cmd/1 -> Demux3/1
  AZ DT Lugre Fr model/1(FrTorque) -> Terminator/1
  EL DT Lugre Fr model/1(FrTorque) -> Terminator1/1
  GIR DT Lugre Fr model/1(FrTorque) -> Terminator2/1

== system ltao_e2e/OIWFS integration ==
  gTT_FP : Inport
  Discrete-Time Integrator : DiscreteIntegrator  gainval=1  ExternalReset=rising  SampleTime=-1  ICPrevOutput=DiscIntNeverNeededParam  ICPrevScaledInput=DiscIntNeverNeededParam
  Mux1 : Mux  Commented=on  Inputs=2
  Pulse Generator : DiscretePulseGenerator  Period=st.ltao.T/fem.Ts  PulseWidth=2  PhaseDelay=1  SampleTime=fem.Ts
  TEST Scope : Scope  Commented=on
  wfs_int_gain : Gain  Gain=1/st.ltao.T
  gTT_WFS : Outport
  wires:
  Pulse Generator/1 -> Discrete-Time Integrator/2
  Discrete-Time Integrator/1 -> wfs_int_gain/1
  Mux1/1 -> TEST Scope/1
  wfs_int_gain/1 -> gTT_WFS/1, Mux1/2
  gTT_FP/1 -> Mux1/1, Discrete-Time Integrator/1

== system ltao_e2e/Segment TT ==
  "M1M2_RBM " : Inport
  LOS Selector : Subsystem  Commented=on
  Seg TT avg removal : Gain  Gain=(eye(14) - kron(eye(2),kron(ones(7),1/7)))  Multiplication=Matrix(K*u)
  Seg TT optical sensitivity matrix : Gain  Gain=D_seg_tt  Multiplication=Matrix(K*u)
  X-Y Motion Error (arcsec) : Scope  Commented=on  NumInputPorts=2
  segTT_FP : Outport  VectorParamsAs1DForOutWhenUnconnected=off
  wires:
  LOS Selector/2(LOS Y) -> X-Y Motion Error (arcsec)/2
  LOS Selector/1(LOS X) -> X-Y Motion Error (arcsec)/1
  "M1M2_RBM "/1 -> Seg TT optical sensitivity matrix/1
  Seg TT optical sensitivity matrix/1 -> Seg TT avg removal/1
  Seg TT avg removal/1 -> segTT_FP/1

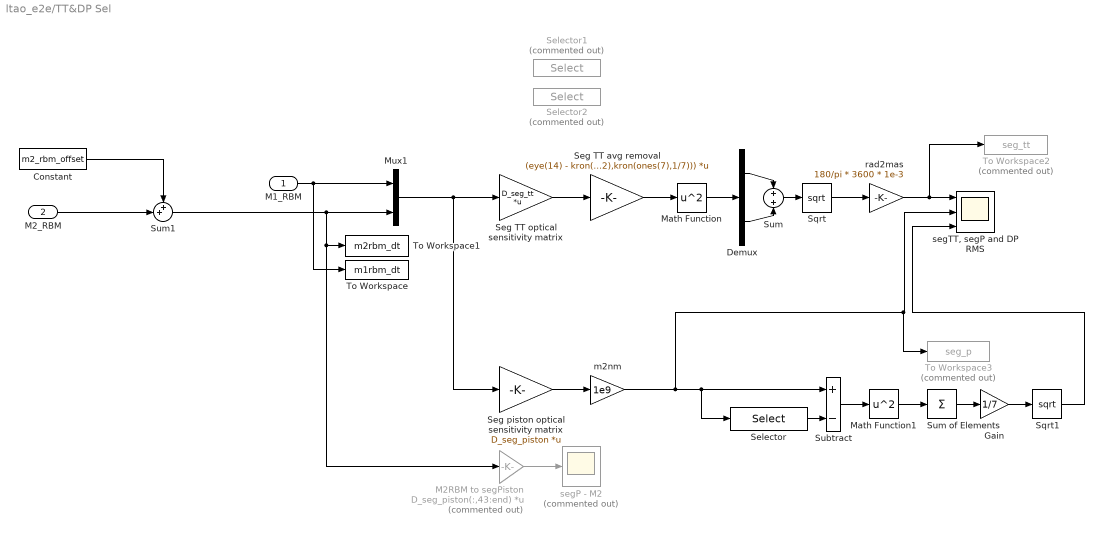
== system ltao_e2e/TT&DP Sel ==
  M1_RBM : Inport
  M2_RBM : Inport  Port=2
  Constant : Constant  Value=m2_rbm_offset
  Demux : Demux  Outputs=[7,7]
  Gain : Gain  Gain=1/7
  M2RBM to segPiston : Gain  Commented=on  Gain=D_seg_piston(:,43:end)  Multiplication=Matrix(K*u)
  Math Function : Math  Operator=square
  Math Function1 : Math  Operator=square
  Mux1 : Mux  Inputs=[42 42]
  Seg TT avg removal : Gain  Gain=(eye(14) - kron(eye(2),kron(ones(7),1/7)))  Multiplication=Matrix(K*u)
  Seg TT optical sensitivity matrix : Gain  Gain=D_seg_tt  Multiplication=Matrix(K*u)
  Seg piston optical sensitivity matrix : Gain  Gain=D_seg_piston  Multiplication=Matrix(K*u)
  Selector : Selector  InputPortWidth=7  IndexOptions=Index vector (dialog)  Indices=[7]  OutputSizes=1
  Selector1 : Selector  Commented=on  InputPortWidth=14  IndexOptions=Index vector (dialog)  Indices=[1:7]  OutputSizes=1
  Selector2 : Selector  Commented=on  InputPortWidth=14  IndexOptions=Index vector (dialog)  Indices=[8:14]  OutputSizes=1
  Sqrt : Sqrt
  Sqrt1 : Sqrt
  Subtract : Sum  Inputs=+-
  Sum : Sum  Inputs=+|+
  Sum of Elements : Sum  Inputs=+
  Sum1 : Sum  Inputs=++|
  To Workspace : ToWorkspace  VariableName=m1rbm_dt  SampleTime=-1
  To Workspace1 : ToWorkspace  VariableName=m2rbm_dt  SampleTime=-1
  To Workspace2 : ToWorkspace  Commented=on  VariableName=seg_tt  SampleTime=-1
  To Workspace3 : ToWorkspace  Commented=on  VariableName=seg_p  SampleTime=-1
  m2nm : Gain  Gain=1e9
  rad2mas : Gain  Gain=180/pi * 3600 * 1e-3
  segP - M2 : Scope  Commented=on
  "segTT, segP and DP RMS" : Scope  NumInputPorts=3
  wires:
  Math Function/1 -> Demux/1
  Demux/1 -> Sum/1
  Demux/2 -> Sum/2
  Sum/1 -> Sqrt/1
  Sqrt/1 -> rad2mas/1
  rad2mas/1 -> To Workspace2/1, "segTT, segP and DP RMS"/1
  Mux1/1 -> Seg piston optical sensitivity matrix/1, Seg TT optical sensitivity matrix/1
  Seg piston optical sensitivity matrix/1 -> m2nm/1
  Sum1/1 -> M2RBM to segPiston/1, To Workspace1/1, Mux1/2
  M1_RBM/1 -> To Workspace/1, Mux1/1
  Seg TT optical sensitivity matrix/1 -> Seg TT avg removal/1
  m2nm/1 -> To Workspace3/1, "segTT, segP and DP RMS"/2, Selector/1, Subtract/1
  Selector/1 -> Subtract/2
  Subtract/1 -> Math Function1/1
  Math Function1/1 -> Sum of Elements/1
  Sum of Elements/1 -> Gain/1
  Gain/1 -> Sqrt1/1
  Sqrt1/1 -> "segTT, segP and DP RMS"/3
  M2RBM to segPiston/1 -> segP - M2/1
  Seg TT avg removal/1 -> Math Function/1
  M2_RBM/1 -> Sum1/2
  Constant/1 -> Sum1/1

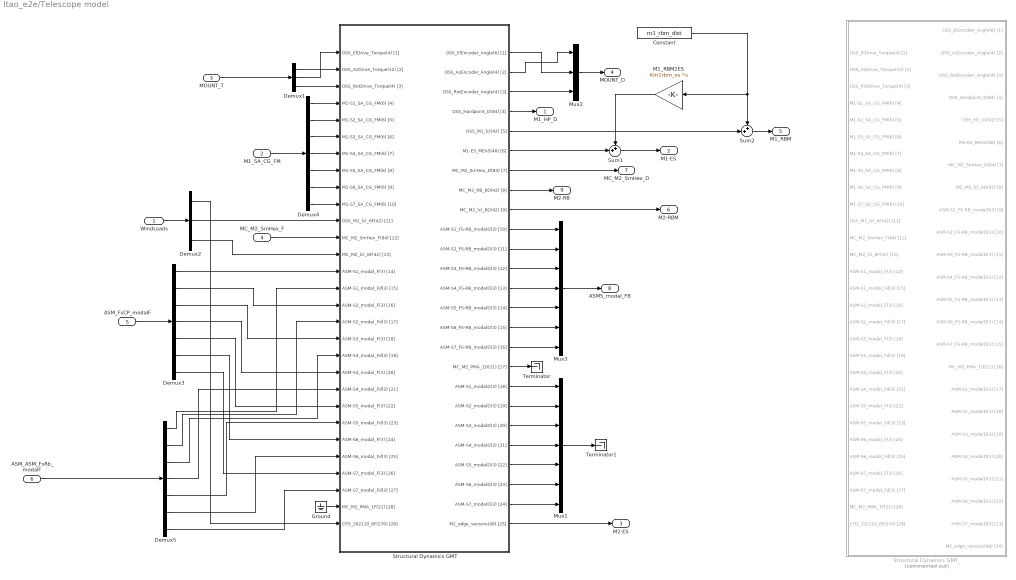
== system ltao_e2e/Telescope model ==
  WindLoads : Inport
  M1_SA_CG_FM : Inport  Port=2
  MOUNT_T : Inport  Port=3
  MC_M2_SmHex_F : Inport  Port=4
  ASM_FsCP_modalF : Inport  Port=5
  ASM_ASM_FsRb_modalF : Inport  Port=6
  Constant : Constant  Value=m1_rbm_dist
  Demux1 : Demux  Outputs=[12,4,4]
  Demux2 : Demux  Outputs=wl_demux
  Demux3 : Demux  Outputs=7
  Demux4 : Demux  Outputs=6*ones(1,7)
  Demux5 : Demux  Outputs=size(asm_ssG,1)*ones(1,7)
  Ground : Ground
  M1_RBM2ES : Gain  Gain=Km1rbm_es  Multiplication=Matrix(K*u) (u vector)
  Mux1 : Mux  Inputs=7
  Mux2 : Mux  Inputs=[4,6,4]
  Mux3 : Mux  Inputs=7
  Structural Dynamics GMT : Subsystem
  Structural Dynamics GMT_ : Subsystem  Commented=on
  Sum1 : Sum  Inputs=++|
  Sum2 : Sum  Inputs=++|
  Terminator : Terminator
  Terminator1 : Terminator
  M1_HP_D : Outport  VectorParamsAs1DForOutWhenUnconnected=off
  M1-ES : Outport  Port=2  VectorParamsAs1DForOutWhenUnconnected=off
  M2-ES : Outport  Port=3  VectorParamsAs1DForOutWhenUnconnected=off
  MOUNT_D : Outport  Port=4  VectorParamsAs1DForOutWhenUnconnected=off
  M1_RBM : Outport  Port=5  VectorParamsAs1DForOutWhenUnconnected=off
  M2-RBM : Outport  Port=6  VectorParamsAs1DForOutWhenUnconnected=off
  MC_M2_SmHex_D : Outport  Port=7  VectorParamsAs1DForOutWhenUnconnected=off
  ASMS_modal_FB : Outport  Port=8  VectorParamsAs1DForOutWhenUnconnected=off
  M2-RB : Outport  Port=9  VectorParamsAs1DForOutWhenUnconnected=off
  wires:
  Demux4/3 -> Structural Dynamics GMT/6(M1-S3_SA_CG_FM(6) [6])
  Demux1/3 -> Structural Dynamics GMT/3(OSS_RotDrive_Torque(4) [3])
  Structural Dynamics GMT/17(MC_M2_PMA_1D(21) [17]) -> Terminator/1
  Demux4/7 -> Structural Dynamics GMT/10(M1-S7_SA_CG_FM(6) [10])
  Demux4/1 -> Structural Dynamics GMT/4(M1-S1_SA_CG_FM(6) [4])
  Demux4/6 -> Structural Dynamics GMT/9(M1-S6_SA_CG_FM(6) [9])
  Structural Dynamics GMT/3(OSS_RotEncoder_Angle(4) [3]) -> Mux2/3
  Demux4/4 -> Structural Dynamics GMT/7(M1-S4_SA_CG_FM(6) [7])
  Demux4/5 -> Structural Dynamics GMT/8(M1-S5_SA_CG_FM(6) [8])
  Demux4/2 -> Structural Dynamics GMT/5(M1-S2_SA_CG_FM(6) [5])
  Structural Dynamics GMT/4(OSS_Hardpoint_D(84) [4]) -> M1_HP_D/1
  Mux1/1 -> Terminator1/1
  Demux1/1 -> Structural Dynamics GMT/2(OSS_AzDrive_Torque(12) [2])
  Demux1/2 -> Structural Dynamics GMT/1(OSS_ElDrive_Torque(4) [1])
  Structural Dynamics GMT/1(OSS_ElEncoder_Angle(6) [1]) -> Mux2/2
  Structural Dynamics GMT/2(OSS_AzEncoder_Angle(4) [2]) -> Mux2/1
  MC_M2_SmHex_F/1 -> Structural Dynamics GMT/12(MC_M2_SmHex_F(84) [12])
  Ground/1 -> Structural Dynamics GMT/28(MC_M2_PMA_1F(21) [28])
  WindLoads/1 -> Demux2/1
  Demux2/1 -> Structural Dynamics GMT/29(CFD_202110_6F(270) [29])
  Demux2/2 -> Structural Dynamics GMT/11(OSS_M1_lcl_6F(42) [11])
  MOUNT_T/1 -> Demux1/1
  Mux2/1 -> MOUNT_D/1
  M1_SA_CG_FM/1 -> Demux4/1
  Demux3/1 -> Structural Dynamics GMT/14(ASM-S1_modal_F(3) [14])
  Demux3/2 -> Structural Dynamics GMT/16(ASM-S2_modal_F(3) [16])
  Demux3/3 -> Structural Dynamics GMT/18(ASM-S3_modal_F(3) [18])
  Demux3/4 -> Structural Dynamics GMT/20(ASM-S4_modal_F(3) [20])
  Demux3/5 -> Structural Dynamics GMT/22(ASM-S5_modal_F(3) [22])
  Demux3/6 -> Structural Dynamics GMT/24(ASM-S6_modal_F(3) [24])
  Demux3/7 -> Structural Dynamics GMT/26(ASM-S7_modal_F(3) [26])
  ASM_FsCP_modalF/1 -> Demux3/1
  Demux5/7 -> Structural Dynamics GMT/27(ASM-S7_modal_Fd(3) [27])
  Demux5/6 -> Structural Dynamics GMT/25(ASM-S6_modal_Fd(3) [25])
  Demux5/5 -> Structural Dynamics GMT/23(ASM-S5_modal_Fd(3) [23])
  Demux5/4 -> Structural Dynamics GMT/21(ASM-S4_modal_Fd(3) [21])
  Demux5/3 -> Structural Dynamics GMT/19(ASM-S3_modal_Fd(3) [19])
  Demux5/2 -> Structural Dynamics GMT/17(ASM-S2_modal_Fd(3) [17])
  Demux5/1 -> Structural Dynamics GMT/15(ASM-S1_modal_Fd(3) [15])
  ASM_ASM_FsRb_modalF/1 -> Demux5/1
  Structural Dynamics GMT/18(ASM-S1_modalD(3) [18]) -> Mux1/1
  Structural Dynamics GMT/19(ASM-S2_modalD(3) [19]) -> Mux1/2
  Structural Dynamics GMT/20(ASM-S3_modalD(3) [20]) -> Mux1/3
  Structural Dynamics GMT/21(ASM-S4_modalD(3) [21]) -> Mux1/4
  Structural Dynamics GMT/22(ASM-S5_modalD(3) [22]) -> Mux1/5
  Structural Dynamics GMT/23(ASM-S6_modalD(3) [23]) -> Mux1/6
  Structural Dynamics GMT/24(ASM-S7_modalD(3) [24]) -> Mux1/7
  Structural Dynamics GMT/16(ASM-S7_FS-RB_modalD(3) [16]) -> Mux3/7
  Structural Dynamics GMT/15(ASM-S6_FS-RB_modalD(3) [15]) -> Mux3/6
  Mux3/1 -> ASMS_modal_FB/1
  Structural Dynamics GMT/7(MC_M2_SmHex_D(84) [7]) -> MC_M2_SmHex_D/1
  Structural Dynamics GMT/14(ASM-S5_FS-RB_modalD(3) [14]) -> Mux3/5
  Structural Dynamics GMT/13(ASM-S4_FS-RB_modalD(3) [13]) -> Mux3/4
  Structural Dynamics GMT/12(ASM-S3_FS-RB_modalD(3) [12]) -> Mux3/3
  Structural Dynamics GMT/11(ASM-S2_FS-RB_modalD(3) [11]) -> Mux3/2
  Structural Dynamics GMT/10(ASM-S1_FS-RB_modalD(3) [10]) -> Mux3/1
  Structural Dynamics GMT/9(MC_M2_lcl_6D(42) [9]) -> M2-RBM/1
  Structural Dynamics GMT/5(OSS_M1_lcl(42) [5]) -> Sum2/2
  Sum2/1 -> M1_RBM/1
  Sum1/1 -> M1-ES/1
  Constant/1 -> M1_RBM2ES/1, Sum2/1
  M1_RBM2ES/1 -> Sum1/1
  Structural Dynamics GMT/6(M1-ES_MEAS(48) [6]) -> Sum1/2
  Structural Dynamics GMT/8(MC_M2_RB_6D(42) [8]) -> M2-RB/1
  Demux2/3 -> Structural Dynamics GMT/13(MC_M2_lcl_6F(42) [13])
  Structural Dynamics GMT/25(M2_edge_sensors(48) [25]) -> M2-ES/1

== system ltao_e2e/Wind Loads ==
  note: Red are the IM wind load time series
  Constant : Constant  Value=osim.bpless_wl
  Mux : Mux  Inputs=2
  Product : Product
  Selector : Selector  InputPortWidth=354  IndexOptions=Index vector (dialog)  Indices=[270+(4:5)]  OutputSizes=1
  Selector1 : Selector  InputPortWidth=354  IndexOptions=Index vector (dialog)  Indices=[270+(4:5)]  OutputSizes=1
  Sigmoid : Subsystem
  Switch : Switch  Criteria=u2 > Threshold  SaturateOnIntegerOverflow=off  InputSameDT=off
  b2021_WL : FromWorkspace  VariableName=IMLoads  SampleTime=-1  OutputAfterFinalValue=Holding final value
  wl_scope : Scope
  wload_en : Gain  Gain=osim.wload_en
  wloads : Outport  VectorParamsAs1DForOutWhenUnconnected=off
  wires:
  wload_en/1 -> Selector1/1, wloads/1
  b2021_WL/1 -> Selector/1, Switch/3, Product/1
  Sigmoid/1(s) -> Product/2
  Product/1 -> Switch/1
  Switch/1 -> wload_en/1
  Constant/1 -> Switch/2
  Selector/1 -> Mux/1
  Selector1/1 -> Mux/2
  Mux/1 -> wl_scope/1

== system ltao_e2e/gTT Controller ==
  note: AO FB compensator 4kHz
  gTT_FB : Inport  PortDimensions=size(rbm2gtt,1)
  C_AO 4kHz : DiscreteTransferFcn  Numerator=fao_d4k.num{1}  Denominator=fao_d4k.den{1}  SampleTime=fao_d4k.Ts
  Ground : Ground
  Mux1 : Mux  Commented=on  Inputs=3
  RT_AO4k : RateTransition  Integrity=off  Deterministic=off  OutPortSampleTimeOpt=Inherit
  RT_ASM : RateTransition  Integrity=off  Deterministic=off  OutPortSampleTimeOpt=Inherit
  Scope : Scope
  Scope1 : Scope  Commented=on
  Selector2 : Selector  Commented=on  InputPortWidth=462  IndexOptions=Index vector (dialog)  Indices=[1 4]  OutputSizes=1
  Selector4 : Selector  Commented=on  InputPortWidth=462  IndexOptions=Index vector (dialog)  Indices=[1 4]  OutputSizes=1
  Selector5 : Selector  Commented=on  InputPortWidth=462  IndexOptions=Index vector (dialog)  Indices=[1 4]  OutputSizes=1
  Sum1 : Sum  Inputs=|+-
  gtt_ctrl_en : Gain  Gain=osim.gtt_fb_en
  gtt_to_segTTP : Gain  Gain=[D_seg_tt; D_seg_piston]*Hk_mnt_m1m2*gtt2mnt  Multiplication=Matrix(K*u)
  segPTT2asmCMD : Subsystem
  ASM_cmd : Outport  VectorParamsAs1DForOutWhenUnconnected=off
  wires:
  Ground/1 -> Sum1/1
  Sum1/1 -> RT_AO4k/1
  Selector4/1 -> Mux1/2
  Selector2/1 -> Mux1/1
  Selector5/1 -> Mux1/3
  RT_AO4k/1 -> C_AO 4kHz/1
  C_AO 4kHz/1 -> RT_ASM/1
  Mux1/1 -> Scope1/1
  RT_ASM/1 -> gtt_to_segTTP/1
  segPTT2asmCMD/1(ASM_KL012_CMD) -> ASM_cmd/1
  gtt_to_segTTP/1 -> segPTT2asmCMD/1(segTTP)
  gtt_ctrl_en/1 -> Sum1/2
  gTT_FB/1 -> Scope/1, gtt_ctrl_en/1

== system ltao_e2e/LTWS Controller/segPTT2asmCMD ==
  segTTP : Inport
  Mux : Mux  Inputs=7
  PTT2ASM_S1 : Gain  Gain=segPTT2asmCMD{1}  Multiplication=Matrix(K*u)
  PTT2ASM_S2 : Gain  Gain=segPTT2asmCMD{2}  Multiplication=Matrix(K*u)
  PTT2ASM_S3 : Gain  Gain=segPTT2asmCMD{3}  Multiplication=Matrix(K*u)
  PTT2ASM_S4 : Gain  Gain=segPTT2asmCMD{4}  Multiplication=Matrix(K*u)
  PTT2ASM_S5 : Gain  Gain=segPTT2asmCMD{5}  Multiplication=Matrix(K*u)
  PTT2ASM_S6 : Gain  Gain=segPTT2asmCMD{6}  Multiplication=Matrix(K*u)
  PTT2ASM_S7 : Gain  Gain=segPTT2asmCMD{7}  Multiplication=Matrix(K*u)
  Selector_S1 : Selector  InputPortWidth=21  IndexOptions=Index vector (dialog)  Indices=1:7:21  OutputSizes=1
  Selector_S2 : Selector  InputPortWidth=21  IndexOptions=Index vector (dialog)  Indices=2:7:21  OutputSizes=1
  Selector_S3 : Selector  InputPortWidth=21  IndexOptions=Index vector (dialog)  Indices=3:7:21  OutputSizes=1
  Selector_S4 : Selector  InputPortWidth=21  IndexOptions=Index vector (dialog)  Indices=4:7:21  OutputSizes=1
  Selector_S5 : Selector  InputPortWidth=21  IndexOptions=Index vector (dialog)  Indices=5:7:21  OutputSizes=1
  Selector_S6 : Selector  InputPortWidth=21  IndexOptions=Index vector (dialog)  Indices=6:7:21  OutputSizes=1
  Selector_S7 : Selector  InputPortWidth=21  IndexOptions=Index vector (dialog)  Indices=7:7:21  OutputSizes=1
  ASM_KL012_CMD : Outport
  wires:
  Mux/1 -> ASM_KL012_CMD/1
  PTT2ASM_S7/1 -> Mux/7
  PTT2ASM_S6/1 -> Mux/6
  PTT2ASM_S5/1 -> Mux/5
  PTT2ASM_S3/1 -> Mux/3
  PTT2ASM_S4/1 -> Mux/4
  PTT2ASM_S2/1 -> Mux/2
  Selector_S4/1 -> PTT2ASM_S4/1
  PTT2ASM_S1/1 -> Mux/1
  Selector_S7/1 -> PTT2ASM_S7/1
  Selector_S6/1 -> PTT2ASM_S6/1
  Selector_S3/1 -> PTT2ASM_S3/1
  Selector_S2/1 -> PTT2ASM_S2/1
  Selector_S1/1 -> PTT2ASM_S1/1
  Selector_S5/1 -> PTT2ASM_S5/1
  segTTP/1 -> Selector_S7/1, Selector_S6/1, Selector_S5/1, Selector_S4/1, Selector_S3/1, Selector_S2/1, Selector_S1/1
